simulink model "DEKF"  (R2017b)
settings: Solver=FixedStepDiscrete  StartTime=0.0  StopTime=inf  FixedStep=dt  RelTol=1e-3  EnableMultiTasking=on
PreLoadFcn:
  | % Quest
  | choice = questdlg('Would you like to load an initial dataset to your workspace?', ...
  | 	'Simulink', ...
  | 	'Yes', 'No', 'No');
  | % Handle response
  | switch choice
  |     case 'Yes'
  |         load('Initialization.mat')
  |     case 'No'
  |     clearvars choice
  | end
values from neighbouring files (symbols this model uses):
  Bat_param =     [Initialization.mat]
  Cnoise = 0.000225    [Initialization.mat]    (also in Simulation_DEKF.m; Simulation_EKF.m)
  Cres = 10    [Initialization.mat]    (also in Simulation_DEKF.m; Simulation_EKF.m)
  dt = 0.025    [Initialization.mat]    (also in Simulation_DEKF.m; Simulation_EKF.m)
  Load_power = [0 0.01 0.02 0.03 0.04 0.05 0.06 0.07 0.08 0.09 0.1 0.11 ... (198604 elements, 99302x2)]    [Initialization.mat]
  P_init = [0.64  0  0; 0  0.0625  0; 0  0  0.0625]    [Initialization.mat]    (also in Simulation_DEKF.m = [0.64,  0,      0;               0,     0.0625, 0;          ; Simulation_EKF.m = [0.64,  0,      0;               0,     0.0625, 0;          )
  Q = [1.2328e-09  0  0; 0  5.3216e-11  0; 0  0  0.00017166]    [Initialization.mat]    (also in Simulation_DEKF.m = [1.2328e-09,  0,      0;           0,           5.3216e-11, ; Simulation_EKF.m = [1.2328e-09,  0,      0;           0,           5.3216e-11, )
  Q_par = [1.6936e-15  0; 0  5.6659e-11]    [Initialization.mat]    (also in Simulation_DEKF.m = [1.6936e-15    0;               0             5.6659e-11]; Simulation_EKF.m = [1.6936e-15    0;               0             5.6659e-11])
  R = 0.7733    [Initialization.mat]    (also in Simulation_DEKF.m; Simulation_EKF.m)
  R_par = 0.00072724    [Initialization.mat]    (also in Simulation_DEKF.m; Simulation_EKF.m)
  S_init = [11.56  0; 0  0.0225]    [Initialization.mat]    (also in Simulation_DEKF.m = [11.56 0;               0     0.0225]; Simulation_EKF.m = [11.56 0;               0     0.0225])
  theta_init = [3.4 0.15]    [Initialization.mat]    (also in Simulation_DEKF.m = [ 3.4, 0.15]'; Simulation_EKF.m = [ 3.4, 0.15]')
  Vnoise = 1.1111e-05    [Initialization.mat]    (also in Simulation_DEKF.m; Simulation_EKF.m)
  Vres = 1.5    [Initialization.mat]    (also in Simulation_DEKF.m; Simulation_EKF.m)
  x_init = [0.8 0 0]    [Initialization.mat]    (also in Simulation_DEKF.m = [0.8, 0, 0]'; Simulation_EKF.m = [0.8, 0, 0]')
undefined symbols (not defined in the file or in its folder): gradient, temperature_LTrange
libraries: simulink x4, dspmtrx3 x2, simulink_extras x1
CloseFcn:
  | % Workspace clear quest
  | choice = questdlg('Would you like to clear the workspace while exiting Simulink?', ...
  | 	'Simulink', ...
  | 	'Yes', 'No', 'No');
  | % Handle response
  | switch choice
  |     case 'Yes'
  |         clear
  |     case 'No'
  |     clearvars choice
  | end
settings Model: PauseTimes=5967  Creator=Hildenbrand  LastModifiedBy=ga73fej
settings DataIOCC: LimitDataPoints=on  SaveFormat=Array  SaveOutput=off  SaveTime=off
settings OptimizationCC: LifeSpan=inf
settings DebuggingCC: BlockPriorityViolationMsg=error  SFUnexpectedBacktrackingDiag=warning  SFNoUnconditionalDefaultTransitionDiag=warning  SFExecutionAtInitializationDiag=none
settings HardwareCC: ProdBitPerPointer=32  ProdBitPerSizeT=32  ProdBitPerPtrDiffT=32  ProdLargestAtomicInteger=Long  ProdLargestAtomicFloat=Double  ProdIntDivRoundTo=Undefined  ProdWordSize=32  ProdHWDeviceType=ARM Compatible->ARM Cortex
settings ModelReferenceCC: PropagateSignalLabelsOutOfModel=off
settings SFSimCC: MATLABDynamicMemAlloc=off
settings RTWCC: SystemTargetFile=ert.tlc  GenCodeOnly=on  TemplateMakefile=ert_default_tmf  Toolchain=Linaro Toolchain v4.8
settings CodeAppCC: IgnoreCustomStorageClasses=off  StateflowObjectComments=on
settings ERTTargetCC: MultiwordLength=2048  GenerateSampleERTMain=on  ERTCustomFileTemplate=example_file_process.tlc  ConvertIfToSwitch=off  SuppressUnreachableDefaultCases=off
settings ConfigComp: CovMetricSettings=dw  CovHtmlReporting=on  CovSaveCumulativeToWorkspaceVar=on  CovSaveSingleToWorkspaceVar=on  CovExternalEMLEnable=off

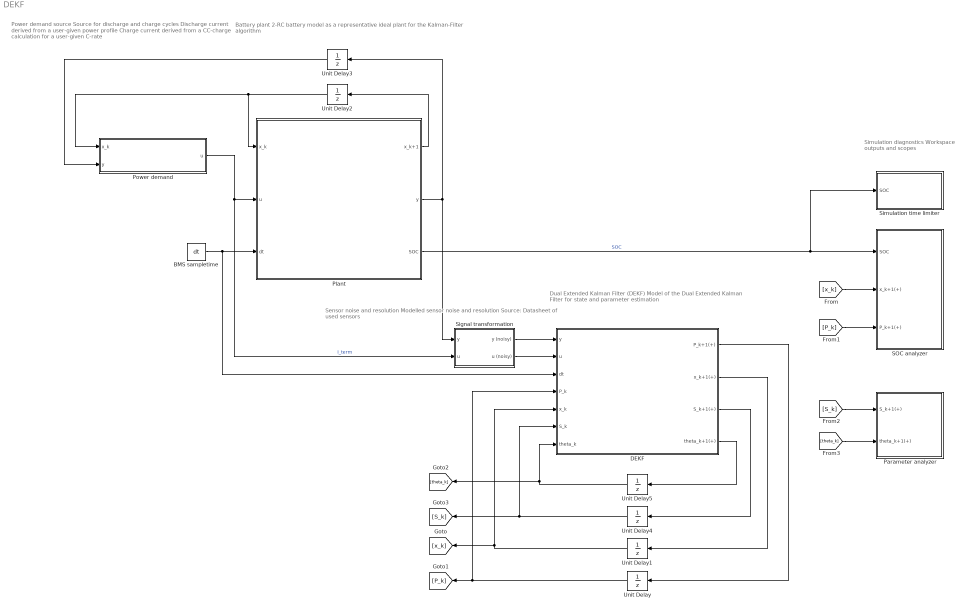
== system DEKF ==
  note: Power demand source
      | Source for discharge and charge cycles
      | Discharge current derived from a user-given power profile
      | Charge current derived from a CC-charge calculation for a user-given C-rate
  note: Battery plant
      | 2-RC battery model as a representative ideal plant
      | for the Kalman-Filter algorithm
  note: Sensor noise and resolution
      | Modelled sensor noise and resolution
      | Source: Datasheet of used sensors
  note: Dual Extended Kalman Filter (DEKF)
      | Model of the Dual Extended Kalman Filter for state and parameter estimation
  note: Simulation diagnostics
      | Workspace outputs and scopes
  BMS sampletime : Constant  Value=dt
  DEKF : Subsystem
  Parameter analyzer : Subsystem
  Plant : Subsystem
  Power demand : Subsystem
  SOC analyzer : Subsystem
  Signal transformation : Subsystem
  Simulation time limiter : Subsystem
  Unit Delay : UnitDelay  InitialCondition=P_init  SampleTime=-1
  Unit Delay1 : UnitDelay  InitialCondition=x_init  SampleTime=-1
  Unit Delay2 : UnitDelay  InitialCondition=Bat_param.Dyn.Bat_init  SampleTime=-1
  Unit Delay3 : UnitDelay  InitialCondition=interp1(Bat_param.Dyn.OCV.SOC,Bat_param.Dyn.OCV.U,Bat_param.Dyn.Bat_init(1))  SampleTime=-1
  Unit Delay4 : UnitDelay  InitialCondition=S_init  SampleTime=-1
  Unit Delay5 : UnitDelay  InitialCondition=theta_init  SampleTime=-1
  wires:
  Power demand/1(u) -> Signal transformation/2(u), Plant/2(u)  "I_term"
  DEKF/1(P_k+1(+)) -> Unit Delay/1
  Unit Delay/1 -> [P_k], DEKF/4(P_k)
  BMS sampletime/1 -> DEKF/3(dt), Plant/3(dt)
  Unit Delay2/1 -> Power demand/1(x_k), Plant/1(x_k)
  Plant/1(x_k+1) -> Unit Delay2/1
  DEKF/3(S_k+1(+)) -> Unit Delay4/1
  Unit Delay4/1 -> [S_k], DEKF/6(S_k)
  DEKF/4(theta_k+1(+)) -> Unit Delay5/1
  Unit Delay5/1 -> [theta_k], DEKF/7(theta_k)
  Plant/2(y) -> Unit Delay3/1, Signal transformation/1(y)
  DEKF/2(x_k+1(+)) -> Unit Delay1/1
  Plant/3(SOC) -> Simulation time limiter/1(SOC), SOC analyzer/1(SOC)  "SOC"
  Unit Delay3/1 -> Power demand/2(y)
  Signal transformation/1(y (noisy)) -> DEKF/1(y)
  Signal transformation/2(u (noisy)) -> DEKF/2(u)
  Unit Delay1/1 -> [x_k], DEKF/5(x_k)
  [x_k] -> SOC analyzer/2(x_k+1(+))
  [P_k] -> SOC analyzer/3(P_k+1(+))
  [S_k] -> Parameter analyzer/1(S_k+1(+))
  [theta_k] -> Parameter analyzer/2(theta_k+1(+))

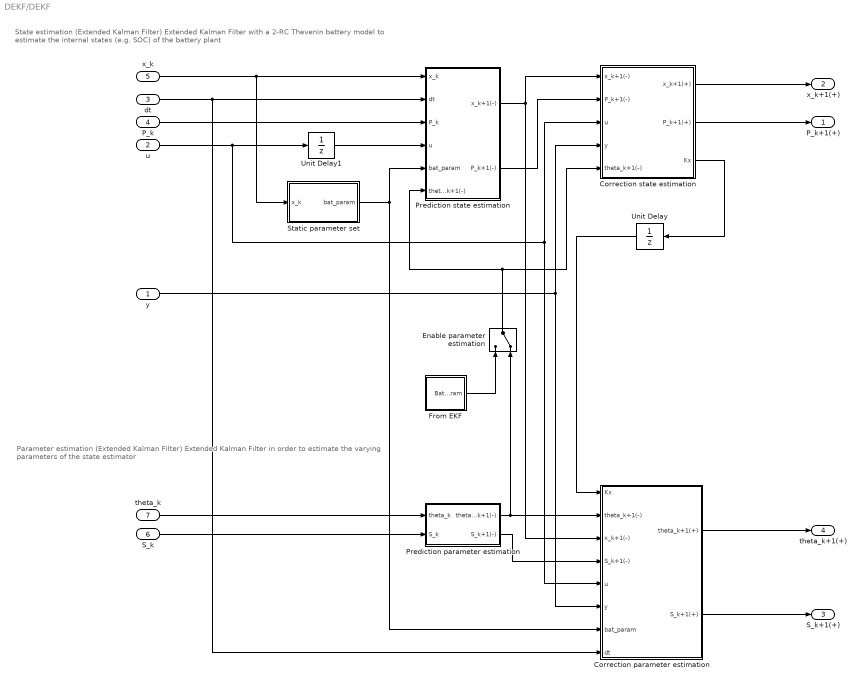
== system DEKF/DEKF ==
  note: State estimation (Extended Kalman Filter)
      | Extended Kalman Filter with a 2-RC Thevenin battery model to estimate the internal states (e.g. SOC) of the battery plant
  note: Parameter estimation (Extended Kalman Filter)
      | Extended Kalman Filter in order to estimate the varying parameters of the state estimator
  y : Inport  PortDimensions=1
  u : Inport  Port=2  PortDimensions=[1 1]
  dt : Inport  Port=3
  P_k : Inport  Port=4
  x_k : Inport  Port=5  PortDimensions=[3 1]
  S_k : Inport  Port=6
  theta_k : Inport  Port=7
  Correction parameter estimation : Subsystem
  Correction state estimation : Subsystem
  Enable parameter estimation : ManualSwitch  CurrentSetting=0
  From EKF : Subsystem
  Prediction parameter estimation : Subsystem
  Prediction state estimation : Subsystem
  "Static parameter set " : Subsystem
  Unit Delay : UnitDelay  InitialCondition=[0; 0; 0]  SampleTime=-1
  Unit Delay1 : UnitDelay  SampleTime=-1
  P_k+1(+) : Outport
  x_k+1(+) : Outport  Port=2
  S_k+1(+) : Outport  Port=3
  theta_k+1(+) : Outport  Port=4
  wires:
  Prediction state estimation/1(x_k+1(-)) -> Correction state estimation/1(x_k+1(-)), Correction parameter estimation/3(x_k+1(-))
  Prediction state estimation/2(P_k+1(-)) -> Correction state estimation/2(P_k+1(-))
  x_k/1 -> "Static parameter set "/1(x_k), Prediction state estimation/1(x_k)
  P_k/1 -> Prediction state estimation/3(P_k)
  y/1 -> Correction state estimation/4(y), Correction parameter estimation/6(y)
  Correction state estimation/2(P_k+1(+)) -> P_k+1(+)/1
  "Static parameter set "/1(bat_param) -> Correction parameter estimation/7(bat_param), Prediction state estimation/5(bat_param)
  dt/1 -> Prediction state estimation/2(dt), Correction parameter estimation/8(dt)
  Correction state estimation/1(x_k+1(+)) -> x_k+1(+)/1
  u/1 -> Correction state estimation/3(u), Correction parameter estimation/5(u), Unit Delay1/1
  Prediction parameter estimation/2(S_k+1(-)) -> Correction parameter estimation/4(S_k+1(-))
  Correction parameter estimation/1(theta_k+1(+)) -> theta_k+1(+)/1
  Correction parameter estimation/2(S_k+1(+)) -> S_k+1(+)/1
  S_k/1 -> Prediction parameter estimation/2(S_k)
  theta_k/1 -> Prediction parameter estimation/1(theta_k)
  Correction state estimation/3(Kx) -> Unit Delay/1
  Unit Delay/1 -> Correction parameter estimation/1(Kx)
  Unit Delay1/1 -> Prediction state estimation/4(u)
  Prediction parameter estimation/1(theta_k+1(-)) -> Enable parameter estimation/2, Correction parameter estimation/2(theta_k+1(-))
  Enable parameter estimation/1 -> Correction state estimation/5(theta_k+1(-)), Prediction state estimation/6(theta_k+1(-))
  From EKF/1(Bat_param) -> Enable parameter estimation/1

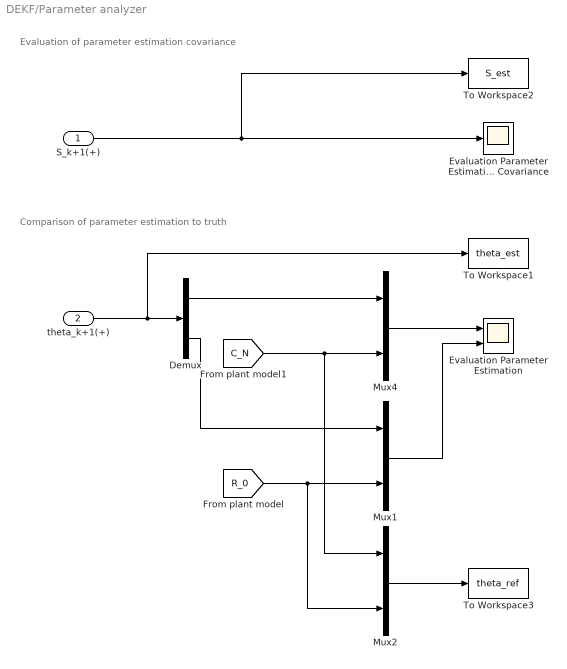
== system DEKF/Parameter analyzer ==
  note: Evaluation of parameter estimation covariance
  note: Comparison of parameter estimation to truth
  S_k+1(+) : Inport
  theta_k+1(+) : Inport  Port=2
  Demux : Demux  Outputs=2
  Evaluation Parameter Estimation : Scope  NumInputPorts=2
  Evaluation Parameter Estimation Covariance : Scope
  Mux1 : Mux  Inputs=2
  Mux2 : Mux  Inputs=2
  Mux4 : Mux  Inputs=2
  To Workspace1 : ToWorkspace  VariableName=theta_est  SaveFormat=Structure With Time  SampleTime=-1
  To Workspace2 : ToWorkspace  VariableName=S_est  SaveFormat=Structure With Time  SampleTime=-1
  To Workspace3 : ToWorkspace  VariableName=theta_ref  SaveFormat=Structure With Time  SampleTime=-1
  wires:
  Demux/1 -> Mux4/1
  Mux4/1 -> Evaluation Parameter Estimation/1
  [C_N] -> Mux2/1, Mux4/2
  S_k+1(+)/1 -> To Workspace2/1, Evaluation Parameter Estimation Covariance/1
  theta_k+1(+)/1 -> To Workspace1/1, Demux/1
  Mux1/1 -> Evaluation Parameter Estimation/2
  [R_0] -> Mux2/2, Mux1/2
  Demux/2 -> Mux1/1
  Mux2/1 -> To Workspace3/1

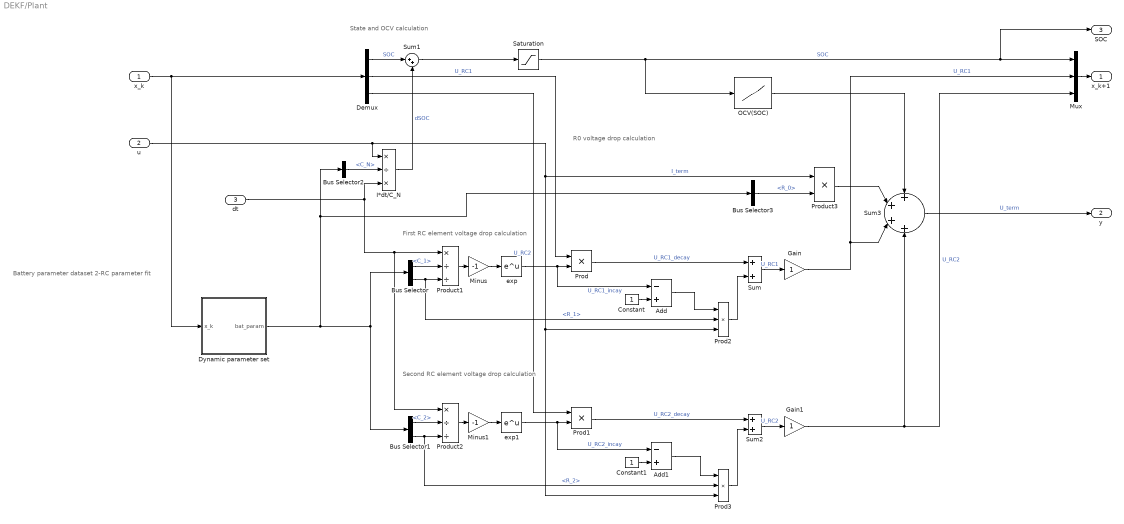
== system DEKF/Plant ==
  note: R0 voltage drop calculation
  note: State and OCV calculation
  note: First RC element voltage drop calculation
  note: Second RC element voltage drop calculation
  note: Battery parameter dataset
      | 2-RC parameter fit
  x_k : Inport  PortDimensions=[3 1]
  u : Inport  Port=2  PortDimensions=[1 1]
  dt : Inport  Port=3
  Add : Sum  Inputs=-+
  Add1 : Sum  Inputs=-+
  Bus Selector : BusSelector  OutputSignals=C_1,R_1
  Bus Selector1 : BusSelector  OutputSignals=C_2,R_2
  Bus Selector2 : BusSelector  OutputSignals=C_N
  Bus Selector3 : BusSelector  OutputSignals=R_0
  Constant : Constant
  Constant1 : Constant
  Demux : Demux  Outputs=3
  Dynamic parameter set : Subsystem
  Gain : Gain
  Gain1 : Gain
  I*dt/C_N : Product  Inputs=*/*
  Minus : Gain  Gain=-1
  Minus1 : Gain  Gain=-1
  Mux : Mux  Inputs=3
  OCV(SOC) : Lookup_n-D  NumberOfTableDimensions=1  BreakpointsForDimension1=Bat_param.Dyn.OCV.SOC  Table=Bat_param.Dyn.OCV.U  ExtrapMethod=Clip  UseLastTableValue=on  InternalRulePriority=Speed  RndMeth=Simplest  InputSameDT=on
  Prod : Product  Inputs=**
  Prod1 : Product  Inputs=**
  Prod2 : Product  Inputs=***
  Prod3 : Product  Inputs=***
  Product1 : Product  Inputs=*//
  Product2 : Product  Inputs=*//
  Product3 : Product  Inputs=**
  Saturation : Saturate  UpperLimit=1  LowerLimit=0
  Sum : Sum
  Sum1 : Sum  Inputs=|++
  Sum2 : Sum
  Sum3 : Sum  Inputs=++++
  exp : Math  SaturateOnIntegerOverflow=on
  exp1 : Math  SaturateOnIntegerOverflow=on
  x_k+1 : Outport
  y : Outport  Port=2
  SOC : Outport  Port=3
  wires:
  Demux/1 -> Sum1/1  "SOC"
  I*dt/C_N/1 -> Sum1/2  "dSOC"
  u/1 -> Prod3/3, Prod2/3, Product3/1, I*dt/C_N/1  "I_term"
  Sum1/1 -> Saturation/1
  Saturation/1 -> SOC/1, Mux/1, OCV(SOC)/1  "SOC"
  Demux/2 -> Prod/1  "U_RC1"
  Dynamic parameter set/1(bat_param) -> Bus Selector2/1, Bus Selector3/1, Bus Selector/1, Bus Selector1/1
  Bus Selector/1 -> Product1/2  "<C_1>"
  Bus Selector/2 -> Prod2/2, Product1/3  "<R_1>"
  Product1/1 -> Minus/1
  Minus/1 -> exp/1
  exp/1 -> Add/1, Prod/2  "U_RC1_incay"
  dt/1 -> Product2/1, Product1/1, I*dt/C_N/3
  Bus Selector1/1 -> Product2/2  "<C_2>"
  Bus Selector1/2 -> Prod3/2, Product2/3  "<R_2>"
  Product2/1 -> Minus1/1
  Minus1/1 -> exp1/1
  exp1/1 -> Add1/1, Prod1/2  "U_RC2_incay"
  Demux/3 -> Prod1/1  "U_RC2"
  Prod1/1 -> Sum2/1  "U_RC2_decay"
  Bus Selector2/1 -> I*dt/C_N/2  "<C_N>"
  Constant/1 -> Add/2
  Constant1/1 -> Add1/2
  Add/1 -> Prod2/1
  Add1/1 -> Prod3/1
  Prod2/1 -> Sum/2
  Prod3/1 -> Sum2/2
  Mux/1 -> x_k+1/1
  Sum/1 -> Gain/1  "U_RC1"
  Sum2/1 -> Gain1/1  "U_RC2"
  Prod/1 -> Sum/1  "U_RC1_decay"
  x_k/1 -> Dynamic parameter set/1(x_k), Demux/1
  Gain/1 -> Mux/2, Sum3/3  "U_RC1"
  Gain1/1 -> Sum3/4, Mux/3  "U_RC2"
  OCV(SOC)/1 -> Sum3/1
  Bus Selector3/1 -> Product3/2  "<R_0>"
  Product3/1 -> Sum3/2
  Sum3/1 -> y/1  "U_term"

== system DEKF/Power demand ==
  note: State switch
      | Charge and Discharge state decision specified by user-defined bounds
  note: Power sources
  x_k : Inport
  y : Inport  Port=2
  Charging Current with specified C-rate : Constant  Value=2.9*0.5
  Lower SOC bound : simulink/Logic and Bit Operations/Compare To Constant  relop=<=  const=0.05  OutDataTypeStr=boolean
  Power profile : simulink/Sources/Repeating Sequence  rep_seq_t=Load_power(:,1)  rep_seq_y=Load_power(:,2)
  Product : Product  Inputs=/*
  S-R Flip-Flop : simulink_extras/Flip Flops/S-R Flip-Flop  initial_condition=1
  Selector3 : Selector  InputPortWidth=3  IndexOptions=Index vector (dialog)  Indices=1  OutputSizes=1
  Switch : Switch  Criteria=u2 > Threshold
  Terminator : Terminator
  Upper SOC bound : simulink/Logic and Bit Operations/Compare To Constant  relop=>=  const=1  OutDataTypeStr=boolean
  u : Outport
  wires:
  Power profile/1 -> Product/2
  Charging Current with specified C-rate/1 -> Switch/3
  Selector3/1 -> Lower SOC bound/1, Upper SOC bound/1  "soc"
  S-R Flip-Flop/1 -> Switch/2
  Upper SOC bound/1 -> S-R Flip-Flop/1
  Lower SOC bound/1 -> S-R Flip-Flop/2
  x_k/1 -> Selector3/1
  S-R Flip-Flop/2 -> Terminator/1
  Product/1 -> Switch/1
  y/1 -> Product/1
  Switch/1 -> u/1

== system DEKF/SOC analyzer ==
  note: Comparison of state estimation error
  note: Comparison of state estimation to truth
  note: Evaluation of state covariance
  SOC : Inport
  x_k+1(+) : Inport  Port=2
  P_k+1(+) : Inport  Port=3
  Evaluation Error of State Estimation : Scope
  Evaluation State Estimation : Scope
  Evaluation State Estimation Covariance : Scope
  Mux3 : Mux  Inputs=2
  Selector1 : Selector  InputPortWidth=3  IndexOptions=Index vector (dialog)  Indices=[1]  OutputSizes=1
  Selector2 : Selector  NumberOfDimensions=2  InputPortWidth=3  IndexOptions=Index vector (dialog),Index vector (dialog)  Indices=[1],[1]  OutputSizes=1,1
  Sum6 : Sum  Inputs=|+-
  To Workspace1 : ToWorkspace  VariableName=SOC_ref  SaveFormat=Structure With Time  SampleTime=-1
  To Workspace2 : ToWorkspace  VariableName=SOC_est  SaveFormat=Structure With Time  SampleTime=-1
  To Workspace3 : ToWorkspace  VariableName=P_est  SaveFormat=Structure With Time  SampleTime=-1
  wires:
  Mux3/1 -> Evaluation State Estimation/1
  Sum6/1 -> Evaluation Error of State Estimation/1
  Selector1/1 -> To Workspace2/1, Sum6/2, Mux3/2  "Estimated SOC"
  x_k+1(+)/1 -> Selector1/1
  SOC/1 -> Mux3/1, Sum6/1, To Workspace1/1  "Reference SOC"
  P_k+1(+)/1 -> Selector2/1
  Selector2/1 -> Evaluation State Estimation Covariance/1, To Workspace3/1  "Estimated SOC"

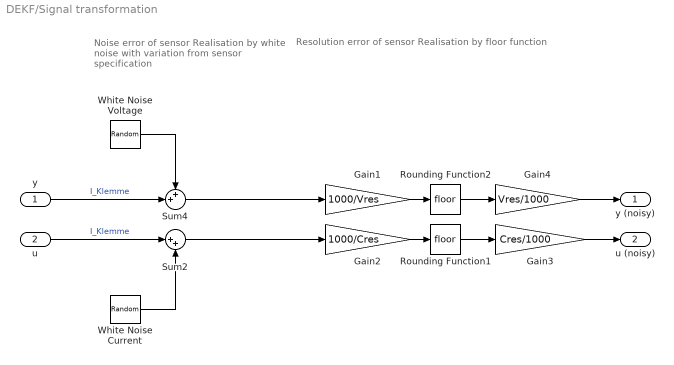
== system DEKF/Signal transformation ==
  note: Resolution error of sensor
      | Realisation by floor function
  note: Noise error of sensor
      | Realisation by white noise
      | with variation from sensor specification
  y : Inport
  u : Inport  Port=2
  Gain1 : Gain  Gain=1000/Vres
  Gain2 : Gain  Gain=1000/Cres
  Gain3 : Gain  Gain=Cres/1000
  Gain4 : Gain  Gain=Vres/1000
  Rounding Function1 : Rounding
  Rounding Function2 : Rounding
  Sum2 : Sum  Inputs=|++
  Sum4 : Sum  Inputs=++|
  White Noise Current : RandomNumber  DisableCoverage=on  Variance=Cnoise  Seed=23341  SampleTime=dt
  White Noise Voltage : RandomNumber  DisableCoverage=on  Variance=Vnoise  Seed=23341  SampleTime=dt
  y (noisy) : Outport
  u (noisy) : Outport  Port=2
  wires:
  Sum4/1 -> Gain1/1
  Sum2/1 -> Gain2/1
  White Noise Current/1 -> Sum2/2
  White Noise Voltage/1 -> Sum4/1
  Gain2/1 -> Rounding Function1/1
  Rounding Function1/1 -> Gain3/1
  Gain1/1 -> Rounding Function2/1
  Rounding Function2/1 -> Gain4/1
  u/1 -> Sum2/1  "I_Klemme"
  Gain3/1 -> u (noisy)/1
  y/1 -> Sum4/2  "I_Klemme"
  Gain4/1 -> y (noisy)/1

== system DEKF/Simulation time limiter ==
  SOC : Inport
  Compare To Constant : simulink/Logic and Bit Operations/Compare To Constant  relop=<=  const=0.1  OutDataTypeStr=boolean
  Stop Simulation : Stop
  wires:
  SOC/1 -> Compare To Constant/1
  Compare To Constant/1 -> Stop Simulation/1

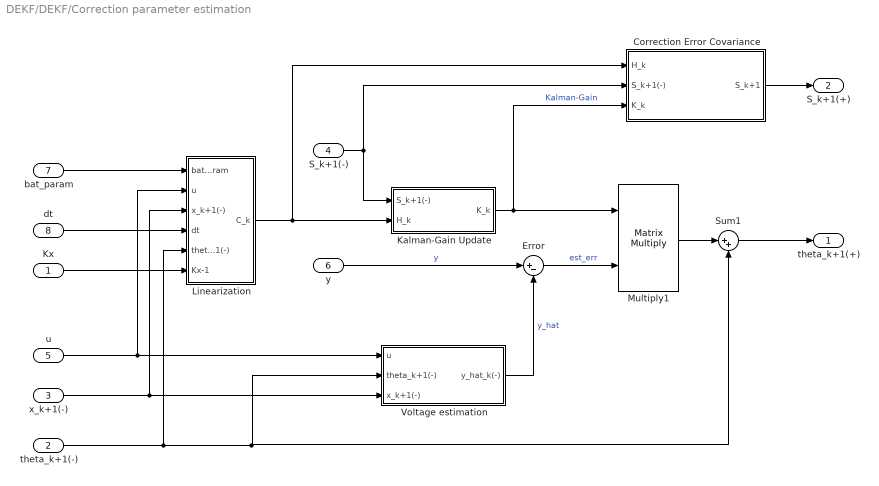
== system DEKF/DEKF/Correction parameter estimation ==
  Kx : Inport
  theta_k+1(-) : Inport  Port=2
  x_k+1(-) : Inport  Port=3
  S_k+1(-) : Inport  Port=4
  u : Inport  Port=5
  y : Inport  Port=6
  bat_param : Inport  Port=7
  dt : Inport  Port=8
  Correction Error Covariance : Subsystem
  Error : Sum  Inputs=|+-
  Kalman-Gain Update : Subsystem
  Linearization : Subsystem
  Multiply1 : Product  Inputs=**  Multiplication=Matrix(*)
  Sum1 : Sum  Inputs=|++
  Voltage estimation : Subsystem
  theta_k+1(+) : Outport
  S_k+1(+) : Outport  Port=2
  wires:
  u/1 -> Linearization/2(u), Voltage estimation/1(u)
  Voltage estimation/1(y_hat_k(-)) -> Error/2  "y_hat"
  S_k+1(-)/1 -> Kalman-Gain Update/1(S_k+1(-)), Correction Error Covariance/2(S_k+1(-))
  Kalman-Gain Update/1(K_k) -> Correction Error Covariance/3(K_k), Multiply1/1  "Kalman-Gain"
  Error/1 -> Multiply1/2  "est_err"
  Multiply1/1 -> Sum1/1
  Sum1/1 -> theta_k+1(+)/1
  Linearization/1(C_k) -> Correction Error Covariance/1(H_k), Kalman-Gain Update/2(H_k)
  Correction Error Covariance/1(S_k+1) -> S_k+1(+)/1
  x_k+1(-)/1 -> Voltage estimation/3(x_k+1(-)), Linearization/3(x_k+1(-))
  y/1 -> Error/1  "y"
  theta_k+1(-)/1 -> Sum1/2, Voltage estimation/2(theta_k+1(-)), Linearization/5(theta_k+1(-))
  Kx/1 -> Linearization/6(Kx-1)
  bat_param/1 -> Linearization/1(bat_param)
  dt/1 -> Linearization/4(dt)

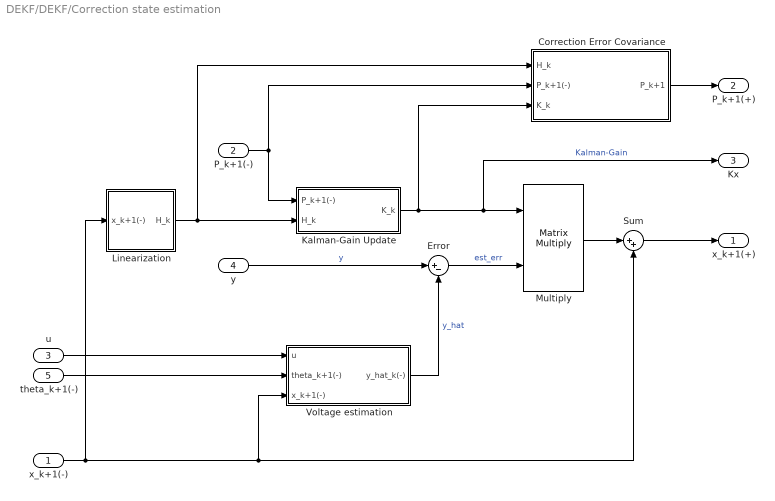
== system DEKF/DEKF/Correction state estimation ==
  x_k+1(-) : Inport
  P_k+1(-) : Inport  Port=2
  u : Inport  Port=3
  y : Inport  Port=4
  theta_k+1(-) : Inport  Port=5
  Correction Error Covariance : Subsystem
  Error : Sum  Inputs=|+-
  Kalman-Gain Update : Subsystem
  Linearization : Subsystem
  Multiply : Product  Inputs=**  Multiplication=Matrix(*)
  Sum : Sum  Inputs=|++
  Voltage estimation : Subsystem
  x_k+1(+) : Outport
  P_k+1(+) : Outport  Port=2
  Kx : Outport  Port=3
  wires:
  u/1 -> Voltage estimation/1(u)
  Voltage estimation/1(y_hat_k(-)) -> Error/2  "y_hat"
  P_k+1(-)/1 -> Kalman-Gain Update/1(P_k+1(-)), Correction Error Covariance/2(P_k+1(-))
  Kalman-Gain Update/1(K_k) -> Correction Error Covariance/3(K_k), Kx/1, Multiply/1  "Kalman-Gain"
  Error/1 -> Multiply/2  "est_err"
  Multiply/1 -> Sum/1
  Sum/1 -> x_k+1(+)/1
  Linearization/1(H_k) -> Correction Error Covariance/1(H_k), Kalman-Gain Update/2(H_k)
  Correction Error Covariance/1(P_k+1) -> P_k+1(+)/1
  x_k+1(-)/1 -> Voltage estimation/3(x_k+1(-)), Sum/2, Linearization/1(x_k+1(-))
  y/1 -> Error/1  "y"
  theta_k+1(-)/1 -> Voltage estimation/2(theta_k+1(-))

== system DEKF/DEKF/From EKF ==
  Mux4 : Mux  Inputs=2
  Bat_param : Outport
  wires:
  [C_N_EKF] -> Mux4/1
  Mux4/1 -> Bat_param/1
  [R_0_EKF] -> Mux4/2

== system DEKF/DEKF/Prediction parameter estimation ==
  theta_k : Inport
  S_k : Inport  Port=2
  Estimation Error Covariance : Subsystem
  State Prediction : Subsystem
  theta_k+1(-) : Outport
  S_k+1(-) : Outport  Port=2
  wires:
  theta_k/1 -> State Prediction/1(theta_k)
  S_k/1 -> Estimation Error Covariance/1(S_k(+))
  State Prediction/1(theta_k+1(-)) -> theta_k+1(-)/1
  Estimation Error Covariance/1(S_k+1(-)) -> S_k+1(-)/1

== system DEKF/DEKF/Prediction state estimation ==
  x_k : Inport
  dt : Inport  Port=2
  P_k : Inport  Port=3  PortDimensions=[3 3]
  u : Inport  Port=4
  bat_param : Inport  Port=5
  theta_k+1(-) : Inport  Port=6
  Estimation Error Covariance : Subsystem
  State Prediction : Subsystem
  x_k+1(-) : Outport
  P_k+1(-) : Outport  Port=2  PortDimensions=[3 3]
  wires:
  x_k/1 -> State Prediction/1(x_k(+))
  u/1 -> State Prediction/2(u)
  P_k/1 -> Estimation Error Covariance/2(P_k(+))
  State Prediction/1(x_k+1(-)) -> x_k+1(-)/1
  Estimation Error Covariance/1(P_k+1(-)) -> P_k+1(-)/1
  bat_param/1 -> State Prediction/4(bat_param), Estimation Error Covariance/3(bat_param)
  dt/1 -> Estimation Error Covariance/1(dt), State Prediction/3(dt)
  theta_k+1(-)/1 -> State Prediction/5(theta_k+1(-))

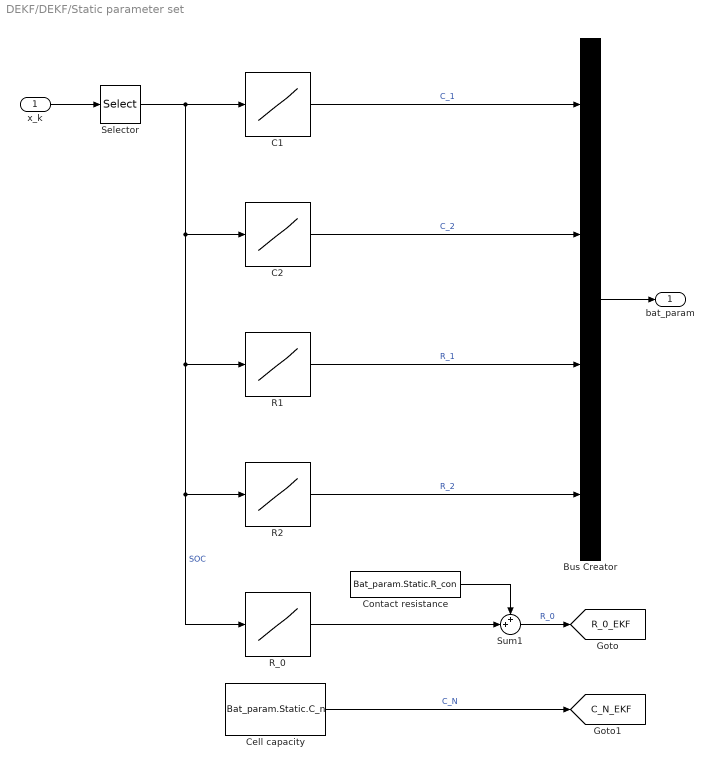
== system DEKF/DEKF/Static parameter set  ==
  x_k : Inport  PortDimensions=[3 1]
  Bus Creator : BusCreator  Inputs=4
  C1 : Lookup_n-D  NumberOfTableDimensions=1  BreakpointsForDimension1=Bat_param.Static.SOC  BreakpointsForDimension2=Bat_param.Static.C_rate  BreakpointsForDimension3=temperature_LTrange  Table=Bat_param.Static.C_1  ExtrapMethod=Clip  UseLastTableValue=on  InternalRulePriority=Speed  RndMeth=Simplest  InputSameDT=on
  C2 : Lookup_n-D  NumberOfTableDimensions=1  BreakpointsForDimension1=Bat_param.Static.SOC  BreakpointsForDimension2=Bat_param.Static.C_rate  BreakpointsForDimension3=temperature_LTrange  Table=Bat_param.Static.C_2  ExtrapMethod=Clip  UseLastTableValue=on  InternalRulePriority=Speed  RndMeth=Simplest  InputSameDT=on
  Cell capacity : Constant  Value=Bat_param.Static.C_n
  Contact resistance : Constant  Value=Bat_param.Static.R_con
  R1 : Lookup_n-D  NumberOfTableDimensions=1  BreakpointsForDimension1=Bat_param.Static.SOC  BreakpointsForDimension2=Bat_param.Static.C_rate  BreakpointsForDimension3=temperature_LTrange  Table=Bat_param.Static.R_1  ExtrapMethod=Clip  UseLastTableValue=on  InternalRulePriority=Speed  RndMeth=Simplest  InputSameDT=on
  R2 : Lookup_n-D  NumberOfTableDimensions=1  BreakpointsForDimension1=Bat_param.Static.SOC  BreakpointsForDimension2=Bat_param.Static.C_rate  BreakpointsForDimension3=temperature_LTrange  Table=Bat_param.Static.R_2  ExtrapMethod=Clip  UseLastTableValue=on  InternalRulePriority=Speed  RndMeth=Simplest  InputSameDT=on
  R_0 : Lookup_n-D  NumberOfTableDimensions=1  BreakpointsForDimension1=Bat_param.Static.SOC  BreakpointsForDimension2=Bat_param.Dyn.C_rate  BreakpointsForDimension3=temperature_LTrange  Table=Bat_param.Static.R_0  ExtrapMethod=Clip  UseLastTableValue=on  InternalRulePriority=Speed  RndMeth=Simplest  InputSameDT=on
  Selector : Selector  InputPortWidth=3  IndexOptions=Index vector (dialog)  Indices=1  OutputSizes=1
  Sum1 : Sum  Inputs=++|
  bat_param : Outport
  tag scope: C_N_EKF=global, R_0_EKF=global
  wires:
  Bus Creator/1 -> bat_param/1
  R1/1 -> Bus Creator/3  "R_1"
  C1/1 -> Bus Creator/1  "C_1"
  R2/1 -> Bus Creator/4  "R_2"
  C2/1 -> Bus Creator/2  "C_2"
  x_k/1 -> Selector/1
  Cell capacity/1 -> [C_N_EKF]  "C_N"
  Contact resistance/1 -> Sum1/1
  Sum1/1 -> [R_0_EKF]  "R_0"
  Selector/1 -> R_0/1, R2/1, R1/1, C2/1, C1/1  "SOC"
  R_0/1 -> Sum1/2

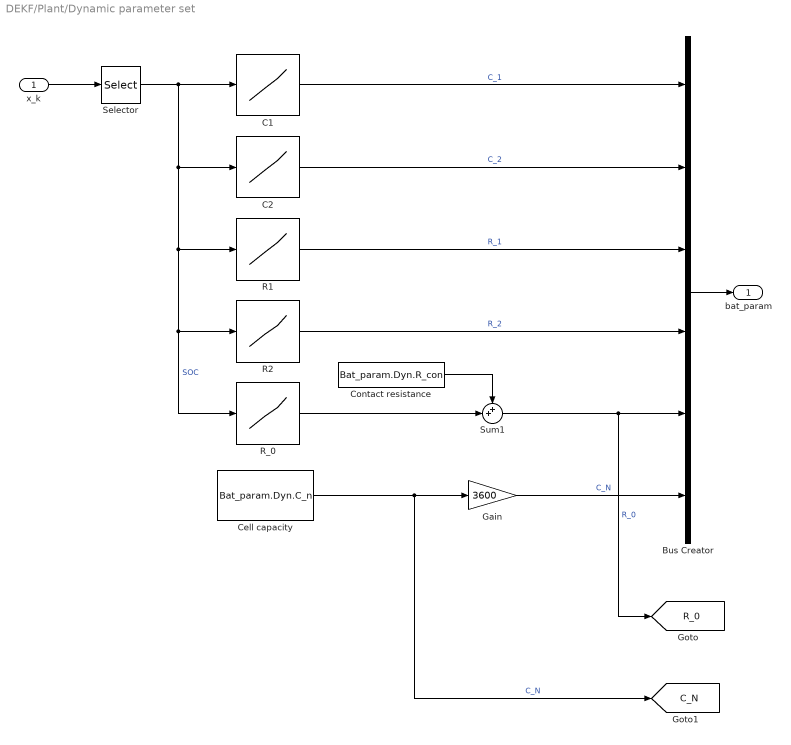
== system DEKF/Plant/Dynamic parameter set ==
  x_k : Inport  PortDimensions=[3 1]
  Bus Creator : BusCreator  Inputs=6
  C1 : Lookup_n-D  NumberOfTableDimensions=1  BreakpointsForDimension1=Bat_param.Dyn.SOC  BreakpointsForDimension2=Bat_param.Dyn.C_rate  BreakpointsForDimension3=temperature_LTrange  Table=Bat_param.Dyn.C_1  ExtrapMethod=Clip  UseLastTableValue=on  InternalRulePriority=Speed  RndMeth=Simplest  InputSameDT=on
  C2 : Lookup_n-D  NumberOfTableDimensions=1  BreakpointsForDimension1=Bat_param.Dyn.SOC  BreakpointsForDimension2=Bat_param.Dyn.C_rate  BreakpointsForDimension3=temperature_LTrange  Table=Bat_param.Dyn.C_2  ExtrapMethod=Clip  UseLastTableValue=on  InternalRulePriority=Speed  RndMeth=Simplest  InputSameDT=on
  Cell capacity : Constant  Value=Bat_param.Dyn.C_n
  Contact resistance : Constant  Value=Bat_param.Dyn.R_con
  Gain : Gain  Gain=3600
  R1 : Lookup_n-D  NumberOfTableDimensions=1  BreakpointsForDimension1=Bat_param.Dyn.SOC  BreakpointsForDimension2=Bat_param.Dyn.C_rate  BreakpointsForDimension3=temperature_LTrange  Table=Bat_param.Dyn.R_1  ExtrapMethod=Clip  UseLastTableValue=on  InternalRulePriority=Speed  RndMeth=Simplest  InputSameDT=on
  R2 : Lookup_n-D  NumberOfTableDimensions=1  BreakpointsForDimension1=Bat_param.Dyn.SOC  BreakpointsForDimension2=Bat_param.Dyn.C_rate  BreakpointsForDimension3=temperature_LTrange  Table=Bat_param.Dyn.R_2  ExtrapMethod=Clip  UseLastTableValue=on  InternalRulePriority=Speed  RndMeth=Simplest  InputSameDT=on
  R_0 : Lookup_n-D  NumberOfTableDimensions=1  BreakpointsForDimension1=Bat_param.Dyn.SOC  BreakpointsForDimension2=Bat_param.Dyn.C_rate  BreakpointsForDimension3=temperature_LTrange  Table=Bat_param.Dyn.R_0  ExtrapMethod=Clip  UseLastTableValue=on  InternalRulePriority=Speed  RndMeth=Simplest  InputSameDT=on
  Selector : Selector  InputPortWidth=3  IndexOptions=Index vector (dialog)  Indices=1  OutputSizes=1
  Sum1 : Sum  Inputs=++|
  bat_param : Outport
  tag scope: C_N=global, R_0=global
  wires:
  Bus Creator/1 -> bat_param/1
  R1/1 -> Bus Creator/3  "R_1"
  Gain/1 -> Bus Creator/6  "C_N"
  C1/1 -> Bus Creator/1  "C_1"
  R2/1 -> Bus Creator/4  "R_2"
  C2/1 -> Bus Creator/2  "C_2"
  R_0/1 -> Sum1/2
  x_k/1 -> Selector/1
  Selector/1 -> R_0/1, R2/1, R1/1, C2/1, C1/1  "SOC"
  Cell capacity/1 -> [C_N], Gain/1  "C_N"
  Sum1/1 -> [R_0], Bus Creator/5  "R_0"
  Contact resistance/1 -> Sum1/1

== system DEKF/DEKF/Correction parameter estimation/Correction Error Covariance ==
  H_k : Inport
  S_k+1(-) : Inport  Port=2
  K_k : Inport  Port=3
  Add : Sum  Inputs=+-
  Multiply : Product  Inputs=**  Multiplication=Matrix(*)
  Multiply1 : Product  Inputs=**  Multiplication=Matrix(*)
  "eye " : Constant  Value=eye(length(theta_init))
  S_k+1 : Outport
  wires:
  S_k+1(-)/1 -> Multiply1/2
  K_k/1 -> Multiply/1
  H_k/1 -> Multiply/2
  Multiply/1 -> Add/2
  Add/1 -> Multiply1/1
  "eye "/1 -> Add/1
  Multiply1/1 -> S_k+1/1

== system DEKF/DEKF/Correction parameter estimation/Kalman-Gain Update ==
  S_k+1(-) : Inport
  H_k : Inport  Port=2
  Add : Sum
  Constant : Constant  Value=R_par
  Multiply : Product  Inputs=***  Multiplication=Matrix(*)
  Multiply1 : Product  Inputs=**  Multiplication=Matrix(*)
  Multiply2 : Product  Inputs=*/  Multiplication=Matrix(*)
  Transpose : Math  Operator=transpose  SaturateOnIntegerOverflow=on
  K_k : Outport
  wires:
  Transpose/1 -> Multiply1/2, Multiply/3
  S_k+1(-)/1 -> Multiply1/1, Multiply/2
  Multiply1/1 -> Multiply2/1
  Add/1 -> Multiply2/2
  Multiply2/1 -> K_k/1
  H_k/1 -> Transpose/1, Multiply/1
  Multiply/1 -> Add/1
  Constant/1 -> Add/2

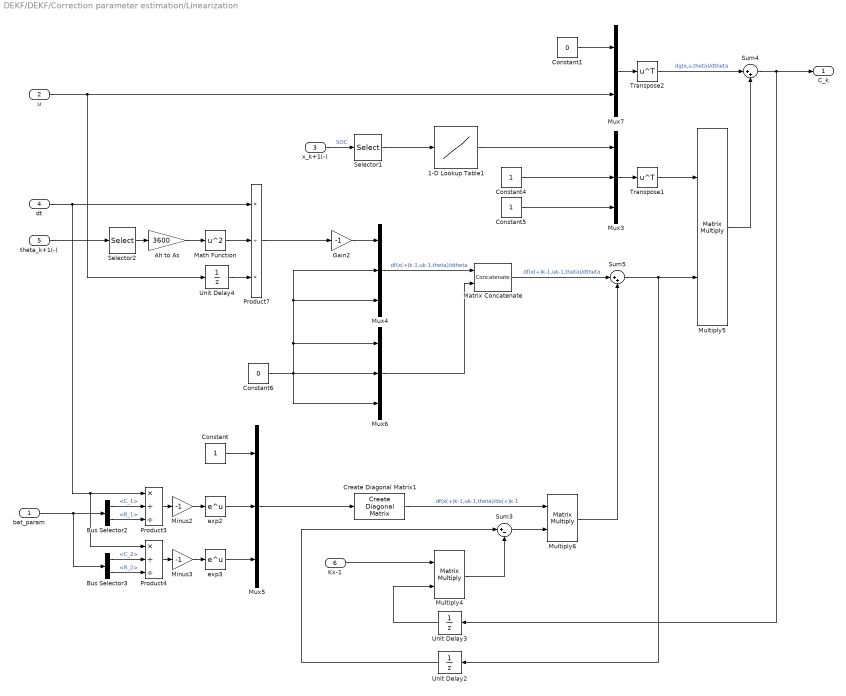
== system DEKF/DEKF/Correction parameter estimation/Linearization ==
  bat_param : Inport
  u : Inport  Port=2
  x_k+1(-) : Inport  Port=3
  dt : Inport  Port=4
  theta_k+1(-) : Inport  Port=5
  Kx-1 : Inport  Port=6
  1-D Lookup Table1 : Lookup_n-D  NumberOfTableDimensions=1  BreakpointsForDimension1=Bat_param.Static.OCV.SOC  Table=(size(Bat_param.Static.OCV.U,2)-1)*gradient(Bat_param.Static.OCV.U)  ExtrapMethod=Clip  UseLastTableValue=on  InternalRulePriority=Speed  RndMeth=Simplest  InputSameDT=on
  Ah to As : Gain  Gain=3600
  Bus Selector2 : BusSelector  OutputSignals=C_1,R_1
  Bus Selector3 : BusSelector  OutputSignals=C_2,R_2
  Constant : Constant
  Constant1 : Constant  Value=0
  Constant4 : Constant
  Constant5 : Constant
  Constant6 : Constant  Value=0
  Create Diagonal Matrix1 : dspmtrx3/Create Diagonal Matrix
      settings: SourceProductName=DSP System Toolbox  SourceProductBaseCode=DS
  Gain2 : Gain  Gain=-1
  Math Function : Math  Operator=square  SaturateOnIntegerOverflow=on
  Matrix Concatenate : Concatenate  Mode=Multidimensional array  ConcatenateDimension=2
  Minus2 : Gain  Gain=-1
  Minus3 : Gain  Gain=-1
  Multiply4 : Product  Inputs=**  Multiplication=Matrix(*)
  Multiply5 : Product  Inputs=**  Multiplication=Matrix(*)
  Multiply6 : Product  Inputs=**  Multiplication=Matrix(*)
  Mux{3..6} (4 alike) : Mux  Inputs=3
  Mux7 : Mux  Inputs=2
  Product3 : Product  Inputs=*//
  Product4 : Product  Inputs=*//
  Product7 : Product  Inputs=*/*
  Selector1 : Selector  InputPortWidth=3  IndexOptions=Index vector (dialog)  Indices=[1]  OutputSizes=1
  Selector2 : Selector  InputPortWidth=2  IndexOptions=Index vector (dialog)  Indices=1  OutputSizes=1
  Sum3 : Sum  Inputs=|+-
  Sum4 : Sum  Inputs=|++
  Sum5 : Sum  Inputs=|++
  Transpose1 : Math  Operator=transpose  SaturateOnIntegerOverflow=on
  Transpose2 : Math  Operator=transpose  SaturateOnIntegerOverflow=on
  Unit Delay2 : UnitDelay  InitialCondition=[0 0; 0 0; 0 0]  SampleTime=-1
  Unit Delay3 : UnitDelay  InitialCondition=[0 0]  SampleTime=-1
  Unit Delay4 : UnitDelay  SampleTime=-1
  exp2 : Math  SaturateOnIntegerOverflow=on
  exp3 : Math  SaturateOnIntegerOverflow=on
  C_k : Outport
  wires:
  Create Diagonal Matrix1/1 -> Multiply6/1  "df(x(+)k-1,uk-1,theta)/dx(+)k-1"
  bat_param/1 -> Bus Selector3/1, Bus Selector2/1
  Bus Selector2/1 -> Product3/2  "<C_1>"
  Bus Selector2/2 -> Product3/3  "<R_1>"
  Product3/1 -> Minus2/1
  Minus2/1 -> exp2/1
  exp2/1 -> Mux5/2
  Bus Selector3/1 -> Product4/2  "<C_2>"
  Bus Selector3/2 -> Product4/3  "<R_2>"
  Product4/1 -> Minus3/1
  Minus3/1 -> exp3/1
  exp3/1 -> Mux5/3
  Constant/1 -> Mux5/1
  Mux5/1 -> Create Diagonal Matrix1/1
  dt/1 -> Product7/1, Product3/1, Product4/1
  Sum4/1 -> C_k/1, Unit Delay3/1
  Mux7/1 -> Transpose2/1
  u/1 -> Mux7/2, Unit Delay4/1
  x_k+1(-)/1 -> Selector1/1  "SOC"
  Math Function/1 -> Product7/2
  Selector2/1 -> Ah to As/1
  Transpose2/1 -> Sum4/1  "dg(x,u,theta)/dtheta"
  Multiply5/1 -> Sum4/2
  Mux3/1 -> Transpose1/1
  1-D Lookup Table1/1 -> Mux3/1
  Constant4/1 -> Mux3/2
  Constant5/1 -> Mux3/3
  Transpose1/1 -> Multiply5/1
  Selector1/1 -> 1-D Lookup Table1/1
  Sum5/1 -> Unit Delay2/1, Multiply5/2
  theta_k+1(-)/1 -> Selector2/1
  Matrix Concatenate/1 -> Sum5/1  "df(x(+)k-1,uk-1,theta)/dtheta"
  Constant6/1 -> Mux4/2, Mux4/3, Mux6/1, Mux6/2, Mux6/3
  Mux4/1 -> Matrix Concatenate/1  "df(x(+)k-1,uk-1,theta)/dtheta"
  Product7/1 -> Gain2/1
  Mux6/1 -> Matrix Concatenate/2
  Gain2/1 -> Mux4/1
  Unit Delay4/1 -> Product7/3
  Ah to As/1 -> Math Function/1
  Multiply6/1 -> Sum5/2
  Sum3/1 -> Multiply6/2
  Unit Delay2/1 -> Sum3/1
  Multiply4/1 -> Sum3/2
  Kx-1/1 -> Multiply4/1
  Unit Delay3/1 -> Multiply4/2
  Constant1/1 -> Mux7/1

== system DEKF/DEKF/Correction parameter estimation/Voltage estimation ==
  u : Inport
  theta_k+1(-) : Inport  Port=2
  x_k+1(-) : Inport  Port=3  PortDimensions=[3 1]
  Demux : Demux  Outputs=3
  OCV(SOC) : Lookup_n-D  NumberOfTableDimensions=1  BreakpointsForDimension1=Bat_param.Static.OCV.SOC  Table=Bat_param.Static.OCV.U  ExtrapMethod=Clip  UseLastTableValue=on  InternalRulePriority=Speed  RndMeth=Simplest  InputSameDT=on
  Product1 : Product  Inputs=**
  Selector2 : Selector  InputPortWidth=2  IndexOptions=Index vector (dialog)  Indices=2  OutputSizes=1
  Sum : Sum  Inputs=++++
  y_hat_k(-) : Outport
  wires:
  Demux/1 -> OCV(SOC)/1  "SOC"
  OCV(SOC)/1 -> Sum/1  "OCV"
  u/1 -> Product1/1  "I_Terminal"
  Sum/1 -> y_hat_k(-)/1  "V_Terminal"
  Demux/2 -> Sum/2  "U_RC1"
  Product1/1 -> Sum/4  "Voltage drop R0"
  x_k+1(-)/1 -> Demux/1
  Demux/3 -> Sum/3  "U_RC2"
  theta_k+1(-)/1 -> Selector2/1
  Selector2/1 -> Product1/2

== system DEKF/DEKF/Correction state estimation/Correction Error Covariance ==
  H_k : Inport
  P_k+1(-) : Inport  Port=2
  K_k : Inport  Port=3
  Add : Sum  Inputs=+-
  Multiply : Product  Inputs=**  Multiplication=Matrix(*)
  Multiply1 : Product  Inputs=**  Multiplication=Matrix(*)
  eye(3) : Constant  Value=eye(3)
  P_k+1 : Outport
  wires:
  P_k+1(-)/1 -> Multiply1/2
  K_k/1 -> Multiply/1
  H_k/1 -> Multiply/2
  Multiply/1 -> Add/2
  Add/1 -> Multiply1/1
  eye(3)/1 -> Add/1
  Multiply1/1 -> P_k+1/1

== system DEKF/DEKF/Correction state estimation/Kalman-Gain Update ==
  P_k+1(-) : Inport
  H_k : Inport  Port=2
  Add : Sum
  Constant : Constant  Value=R
  Multiply : Product  Inputs=***  Multiplication=Matrix(*)
  Multiply1 : Product  Inputs=**  Multiplication=Matrix(*)
  Multiply2 : Product  Inputs=*/  Multiplication=Matrix(*)
  Transpose : Math  Operator=transpose  SaturateOnIntegerOverflow=on
  K_k : Outport
  wires:
  Transpose/1 -> Multiply1/2, Multiply/3
  P_k+1(-)/1 -> Multiply1/1, Multiply/2
  Multiply1/1 -> Multiply2/1
  Add/1 -> Multiply2/2
  Multiply2/1 -> K_k/1
  H_k/1 -> Transpose/1, Multiply/1
  Multiply/1 -> Add/1
  Constant/1 -> Add/2

== system DEKF/DEKF/Correction state estimation/Linearization ==
  x_k+1(-) : Inport
  1-D Lookup Table : Lookup_n-D  NumberOfTableDimensions=1  BreakpointsForDimension1=Bat_param.Static.OCV.SOC  Table=(size(Bat_param.Static.OCV.U,2)-1)*(gradient(Bat_param.Static.OCV.U))  ExtrapMethod=Clip  UseLastTableValue=on  InternalRulePriority=Speed  RndMeth=Simplest  InputSameDT=on
  Constant : Constant
  Constant1 : Constant
  Mux : Mux  Inputs=3
  Selector : Selector  InputPortWidth=3  IndexOptions=Index vector (dialog)  Indices=[1]  OutputSizes=1
  H_k : Outport  PortDimensions=[1 3]
  wires:
  x_k+1(-)/1 -> Selector/1
  Selector/1 -> 1-D Lookup Table/1  "SOC_k"
  1-D Lookup Table/1 -> Mux/1
  Mux/1 -> H_k/1
  Constant/1 -> Mux/2
  Constant1/1 -> Mux/3

== system DEKF/DEKF/Correction state estimation/Voltage estimation ==
  u : Inport
  theta_k+1(-) : Inport  Port=2
  x_k+1(-) : Inport  Port=3  PortDimensions=[3 1]
  Demux : Demux  Outputs=3
  OCV(SOC) : Lookup_n-D  NumberOfTableDimensions=1  BreakpointsForDimension1=Bat_param.Static.OCV.SOC  Table=Bat_param.Static.OCV.U  ExtrapMethod=Clip  UseLastTableValue=on  InternalRulePriority=Speed  RndMeth=Simplest  InputSameDT=on
  Product1 : Product  Inputs=**
  Selector1 : Selector  InputPortWidth=2  IndexOptions=Index vector (dialog)  Indices=2  OutputSizes=1
  Sum : Sum  Inputs=++++
  y_hat_k(-) : Outport
  wires:
  Demux/1 -> OCV(SOC)/1  "SOC"
  OCV(SOC)/1 -> Sum/1  "OCV"
  u/1 -> Product1/1  "I_Terminal"
  Sum/1 -> y_hat_k(-)/1  "V_Terminal"
  Demux/2 -> Sum/2  "U_RC1"
  Product1/1 -> Sum/4  "Voltage drop R0"
  x_k+1(-)/1 -> Demux/1
  Demux/3 -> Sum/3  "U_RC2"
  theta_k+1(-)/1 -> Selector1/1
  Selector1/1 -> Product1/2

== system DEKF/DEKF/Prediction parameter estimation/Estimation Error Covariance ==
  S_k(+) : Inport
  Add : Sum  Inputs=|++
  Covariance Process Noise : Constant  Value=Q_par
  S_k+1(-) : Outport
  wires:
  Covariance Process Noise/1 -> Add/2
  Add/1 -> S_k+1(-)/1
  S_k(+)/1 -> Add/1

== system DEKF/DEKF/Prediction parameter estimation/State Prediction ==
  theta_k : Inport
  theta_k+1(-) : Outport
  wires:
  theta_k/1 -> theta_k+1(-)/1

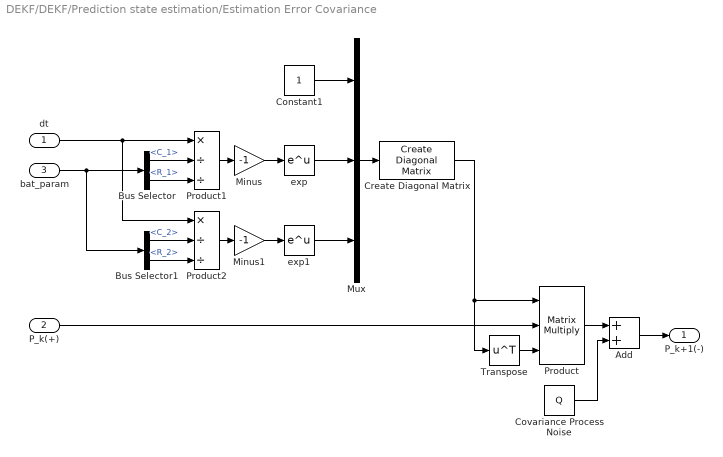
== system DEKF/DEKF/Prediction state estimation/Estimation Error Covariance ==
  dt : Inport
  P_k(+) : Inport  Port=2
  bat_param : Inport  Port=3
  Add : Sum
  Bus Selector : BusSelector  OutputSignals=C_1,R_1
  Bus Selector1 : BusSelector  OutputSignals=C_2,R_2
  Constant1 : Constant
  Covariance Process Noise : Constant  Value=Q
  Create Diagonal Matrix : dspmtrx3/Create Diagonal Matrix
      settings: SourceProductName=DSP System Toolbox  SourceProductBaseCode=DS
  Minus : Gain  Gain=-1
  Minus1 : Gain  Gain=-1
  Mux : Mux  Inputs=3
  Product : Product  Inputs=***  Multiplication=Matrix(*)
  Product1 : Product  Inputs=*//
  Product2 : Product  Inputs=*//
  Transpose : Math  Operator=transpose  SaturateOnIntegerOverflow=on
  exp : Math  SaturateOnIntegerOverflow=on
  exp1 : Math  SaturateOnIntegerOverflow=on
  P_k+1(-) : Outport
  wires:
  P_k(+)/1 -> Product/2
  Transpose/1 -> Product/3
  Create Diagonal Matrix/1 -> Transpose/1, Product/1
  Product/1 -> Add/1
  Covariance Process Noise/1 -> Add/2
  Add/1 -> P_k+1(-)/1
  bat_param/1 -> Bus Selector1/1, Bus Selector/1
  Bus Selector/1 -> Product1/2  "<C_1>"
  Bus Selector/2 -> Product1/3  "<R_1>"
  Product1/1 -> Minus/1
  Minus/1 -> exp/1
  exp/1 -> Mux/2
  dt/1 -> Product2/1, Product1/1
  Bus Selector1/1 -> Product2/2  "<C_2>"
  Bus Selector1/2 -> Product2/3  "<R_2>"
  Product2/1 -> Minus1/1
  Minus1/1 -> exp1/1
  exp1/1 -> Mux/3
  Constant1/1 -> Mux/1
  Mux/1 -> Create Diagonal Matrix/1

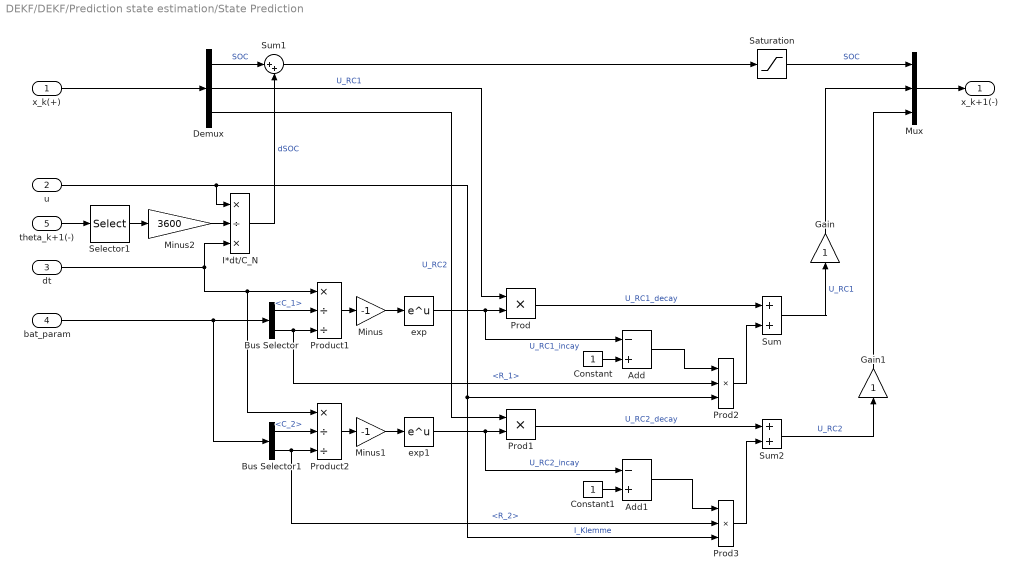
== system DEKF/DEKF/Prediction state estimation/State Prediction ==
  x_k(+) : Inport  PortDimensions=[3 1]
  u : Inport  Port=2  PortDimensions=[1 1]
  dt : Inport  Port=3  PortDimensions=[1 1]
  bat_param : Inport  Port=4
  theta_k+1(-) : Inport  Port=5
  Add : Sum  Inputs=-+
  Add1 : Sum  Inputs=-+
  Bus Selector : BusSelector  OutputSignals=C_1,R_1
  Bus Selector1 : BusSelector  OutputSignals=C_2,R_2
  Constant : Constant
  Constant1 : Constant
  Demux : Demux  Outputs=3
  Gain : Gain
  Gain1 : Gain
  I*dt/C_N : Product  Inputs=*/*
  Minus : Gain  Gain=-1
  Minus1 : Gain  Gain=-1
  Minus2 : Gain  Gain=3600
  Mux : Mux  Inputs=3
  Prod : Product  Inputs=**
  Prod1 : Product  Inputs=**
  Prod2 : Product  Inputs=***
  Prod3 : Product  Inputs=***
  Product1 : Product  Inputs=*//
  Product2 : Product  Inputs=*//
  Saturation : Saturate  UpperLimit=1  LowerLimit=0
  Selector1 : Selector  InputPortWidth=2  IndexOptions=Index vector (dialog)  Indices=[1]  OutputSizes=1
  Sum : Sum
  Sum1 : Sum  Inputs=|++
  Sum2 : Sum
  exp : Math  SaturateOnIntegerOverflow=on
  exp1 : Math  SaturateOnIntegerOverflow=on
  x_k+1(-) : Outport  PortDimensions=[3 1]
  wires:
  x_k(+)/1 -> Demux/1
  Demux/1 -> Sum1/1  "SOC"
  I*dt/C_N/1 -> Sum1/2  "dSOC"
  u/1 -> Prod3/3, Prod2/3, I*dt/C_N/1  "I_Klemme"
  Sum1/1 -> Saturation/1
  Saturation/1 -> Mux/1  "SOC"
  Demux/2 -> Prod/1  "U_RC1"
  bat_param/1 -> Bus Selector1/1, Bus Selector/1
  Bus Selector/1 -> Product1/2  "<C_1>"
  Bus Selector/2 -> Prod2/2, Product1/3  "<R_1>"
  Product1/1 -> Minus/1
  Minus/1 -> exp/1
  exp/1 -> Add/1, Prod/2  "U_RC1_incay"
  dt/1 -> Product2/1, Product1/1, I*dt/C_N/3
  Bus Selector1/1 -> Product2/2  "<C_2>"
  Bus Selector1/2 -> Prod3/2, Product2/3  "<R_2>"
  Product2/1 -> Minus1/1
  Minus1/1 -> exp1/1
  exp1/1 -> Add1/1, Prod1/2  "U_RC2_incay"
  Demux/3 -> Prod1/1  "U_RC2"
  Prod1/1 -> Sum2/1  "U_RC2_decay"
  Constant/1 -> Add/2
  Constant1/1 -> Add1/2
  Add/1 -> Prod2/1
  Add1/1 -> Prod3/1
  Prod2/1 -> Sum/2
  Prod3/1 -> Sum2/2
  Mux/1 -> x_k+1(-)/1
  Sum/1 -> Gain/1  "U_RC1"
  Sum2/1 -> Gain1/1  "U_RC2"
  Prod/1 -> Sum/1  "U_RC1_decay"
  Gain/1 -> Mux/2
  Gain1/1 -> Mux/3
  theta_k+1(-)/1 -> Selector1/1
  Selector1/1 -> Minus2/1
  Minus2/1 -> I*dt/C_N/2
